simulink model "pathFollowingWithObstacleAvoidance"  (R2020a)
settings: Solver=FixedStepDiscrete  StartTime=0.0  StopTime=inf  FixedStep=0.001  RelTol=1e-3
model workspace (MAT data in the model file):
  SL_ROS_VariableLengthArrays_MaxSizes.CommonInfo.ArrayTruncateAction = 'EmitWarning'
  SL_ROS_VariableLengthArrays_MaxSizes.MsgTypeMap = containers.Map
  SL_ROS_VariableLengthArrays_MaxSizes.MsgTypeMap.serialization.keys = {'sensor_msgs/LaserScan'}
  SL_ROS_VariableLengthArrays_MaxSizes.MsgTypeMap.serialization.values{1}(1).PropertyName = 'Intensities'
  SL_ROS_VariableLengthArrays_MaxSizes.MsgTypeMap.serialization.values{1}(1).DataType = 'single'
  SL_ROS_VariableLengthArrays_MaxSizes.MsgTypeMap.serialization.values{1}(1).MaxLength = 360
  SL_ROS_VariableLengthArrays_MaxSizes.MsgTypeMap.serialization.values{1}(2).PropertyName = 'Ranges'
  SL_ROS_VariableLengthArrays_MaxSizes.MsgTypeMap.serialization.values{1}(2).DataType = 'single'
  SL_ROS_VariableLengthArrays_MaxSizes.MsgTypeMap.serialization.values{1}(2).MaxLength = 360
  SL_ROS_VariableLengthArrays_MaxSizes.MsgTypeMap.serialization.uniformity = 0
  SL_ROS_VariableLengthArrays_MaxSizes.MsgTypeMap.serialization.keyType = 'char'
  SL_ROS_VariableLengthArrays_MaxSizes.MsgTypeMap.serialization.valueType = 'any'
undefined symbols (not defined in the file): Angular, Linear
libraries: robotlib x4, robotalgslib x2, sharedtransform x1, simulink x1
settings Model: Creator=Zozo  LastModifiedBy=Zozo
settings OptimizationCC: EnhancedBackFolding=on  PassReuseOutputArgsAs=Individual arguments  ZeroExternalMemoryAtStartup=off  ZeroInternalMemoryAtStartup=off  MaxStackSize=64  OptimizeBlockOrder=speed  DifferentSizesBufferReuse=on  OptimizationCustomize=off  EfficientTunableParamExpr=on
settings DebuggingCC: ParameterTunabilityLossMsg=error
settings HardwareCC: ProdBitPerPointer=32  ProdBitPerSizeT=32  ProdBitPerPtrDiffT=32  ProdLargestAtomicFloat=None  ProdIntDivRoundTo=Undefined  ProdEndianess=Unspecified  ProdWordSize=32  ProdHWDeviceType=Generic->Unspecified (assume 32-bit Generic)
settings SFSimCC: MATLABDynamicMemAlloc=off
settings RTWCC: SystemTargetFile=ert.tlc  HardwareBoard=Robot Operating System (ROS)  TemplateMakefile=ert_default_tmf  Toolchain=Catkin  TargetLang=C++
settings CodeAppCC: ForceParamTrailComments=on  IgnoreCustomStorageClasses=off  OperatorAnnotations=on  SimulinkDataObjDesc=on  SFDataObjDesc=on  InsertBlockDesc=on

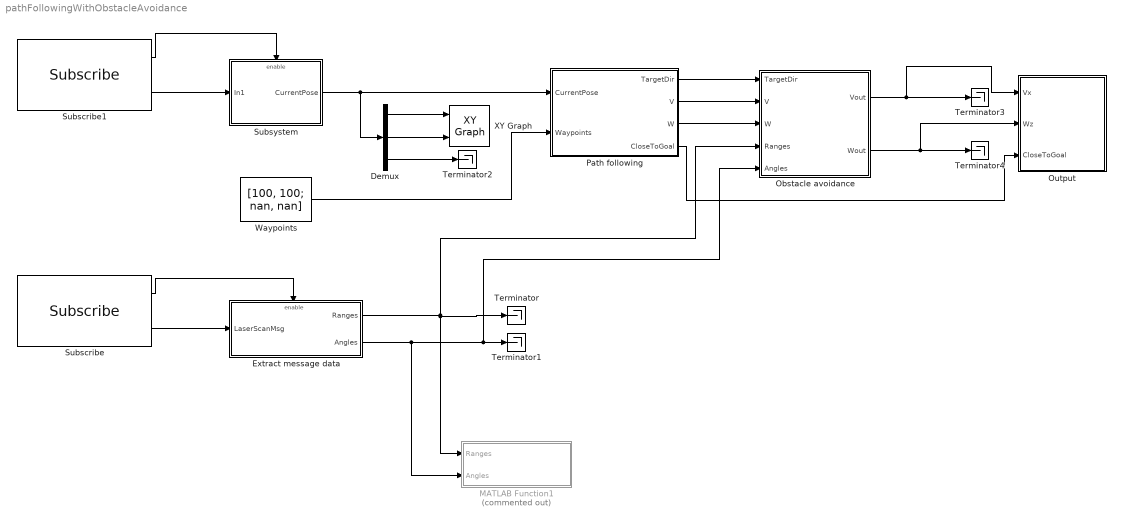
== system pathFollowingWithObstacleAvoidance ==
  Demux : Demux  Outputs=3
  Extract message data : Subsystem
  MATLAB Function1 : MATLAB Function  Commented=on  TreatAsAtomicUnit=on
  Obstacle avoidance : Subsystem
  Output : Subsystem
  Path following : Subsystem
  Subscribe : robotlib/Subscribe  topicSource=Select from ROS network  topic=/lidar2Dscan  messageType=sensor_msgs/LaserScan  sampleTime=-1  messageQueueLength=1
  Subscribe1 : robotlib/Subscribe  topicSource=Select from ROS network  topic=/mavros/local_position/pose  messageType=geometry_msgs/PoseStamped  sampleTime=-1  messageQueueLength=1
  Subsystem : Subsystem
  Terminator{,1..4} (5 alike) : Terminator
  Waypoints : Constant  Value=[100, 100; nan, nan]  OutDataTypeStr=double
  XY Graph : simulink/Sinks/XY Graph  xmin=-10  xmax=30  ymin=-10  ymax=10  st=-1
  wires:
  Subscribe/2 -> Extract message data/1(LaserScanMsg)
  Subscribe/1 -> Extract message data/Enable
  Extract message data/2(Angles) -> Obstacle avoidance/5(Angles), Terminator1/1, MATLAB Function1/2(Angles)
  Extract message data/1(Ranges) -> Terminator/1, MATLAB Function1/1(Ranges), Obstacle avoidance/4(Ranges)
  Subscribe1/2 -> Subsystem/1(In1)
  Subscribe1/1 -> Subsystem/Enable
  Demux/2 -> XY Graph/2
  Demux/1 -> XY Graph/1
  Demux/3 -> Terminator2/1
  Subsystem/1(CurrentPose) -> Path following/1(CurrentPose), Demux/1
  Waypoints/1 -> Path following/2(Waypoints)
  Path following/3(W) -> Obstacle avoidance/3(W)
  Path following/2(V) -> Obstacle avoidance/2(V)
  Path following/1(TargetDir) -> Obstacle avoidance/1(TargetDir)
  Obstacle avoidance/1(Vout) -> Output/1(Vx), Terminator3/1
  Obstacle avoidance/2(Wout) -> Output/2(Wz), Terminator4/1
  Path following/4(CloseToGoal) -> Output/3(CloseToGoal)

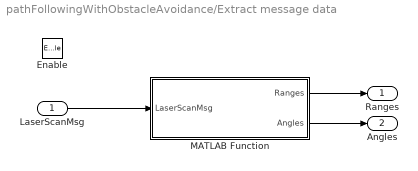
== system pathFollowingWithObstacleAvoidance/Extract message data ==
  LaserScanMsg : Inport
  Enable : EnablePort
  MATLAB Function : MATLAB Function  TreatAsAtomicUnit=on
  Ranges : Outport
  Angles : Outport  Port=2
  wires:
  MATLAB Function/1(Ranges) -> Ranges/1
  MATLAB Function/2(Angles) -> Angles/1
  LaserScanMsg/1 -> MATLAB Function/1(LaserScanMsg)

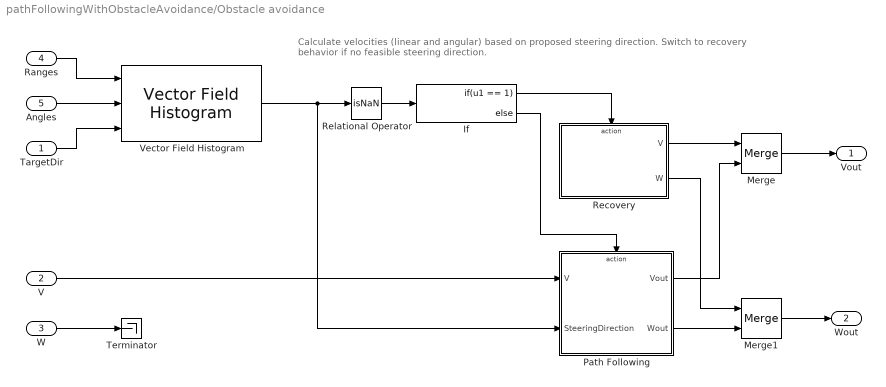
== system pathFollowingWithObstacleAvoidance/Obstacle avoidance ==
  note: Calculate velocities (linear and angular) based on proposed steering direction.
      | 				Switch to recovery behavior if no feasible steering direction.
  TargetDir : Inport
  V : Inport  Port=2
  W : Inport  Port=3
  Ranges : Inport  Port=4
  Angles : Inport  Port=5
  If : If  IfExpression=u1 == 1
  Merge : Merge
  Merge1 : Merge
  Path Following : Subsystem  TreatAsAtomicUnit=on
  Recovery : Subsystem  TreatAsAtomicUnit=on
  Relational Operator : RelationalOperator  Operator=isNaN  OutDataTypeStr=boolean  RndMeth=Simplest
  Terminator : Terminator
  Vector Field Histogram : robotalgslib/Vector Field Histogram  NumAngularSectors=180  DistanceLimits=[0.5, 4]  HistogramThresholds=[3, 10]  RobotRadius=0.25  SafetyDistance=0.25  MinTurningRadius=0.1  SimulateUsing=Code generation  TargetDirectionWeight=5  CurrentDirectionWeight=2  PreviousDirectionWeight=2
      settings: SourceProductBaseCode=RO
  Vout : Outport
  Wout : Outport  Port=2
  wires:
  V/1 -> Path Following/1(V)
  Vector Field Histogram/1 -> Path Following/2(SteeringDirection), Relational Operator/1
  Relational Operator/1 -> If/1
  Angles/1 -> Vector Field Histogram/2
  Merge/1 -> Vout/1
  TargetDir/1 -> Vector Field Histogram/3
  Ranges/1 -> Vector Field Histogram/1
  If/1 -> Recovery/Action
  If/2 -> Path Following/Action
  Recovery/2(W) -> Merge1/1
  Path Following/2(Wout) -> Merge1/2
  Recovery/1(V) -> Merge/1
  Path Following/1(Vout) -> Merge/2
  Merge1/1 -> Wout/1
  W/1 -> Terminator/1

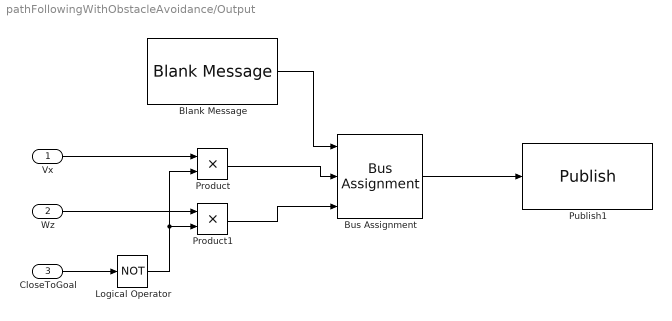
== system pathFollowingWithObstacleAvoidance/Output ==
  Vx : Inport
  Wz : Inport  Port=2
  CloseToGoal : Inport  Port=3
  Blank Message : robotlib/Blank Message  messageClass=Message  entityType=geometry_msgs/Twist  messageType=geometry_msgs/Twist  SampleTime=0
  Bus Assignment : BusAssignment  DialogController=Simulink.DDGSource_BusAssignment  AssignedSignals=Linear.X,Angular.Z
  Logical Operator : Logic  Operator=NOT  AllPortsSameDT=off  OutDataTypeStr=boolean
  Product : Product
  Product1 : Product
  Publish1 : robotlib/Publish  topicSource=Specify your own  topic=/simulink/cmd_vel  messageType=geometry_msgs/Twist  messageQueueLength=105
  wires:
  Bus Assignment/1 -> Publish1/1
  Blank Message/1 -> Bus Assignment/1
  Logical Operator/1 -> Product1/2, Product/2
  Product1/1 -> Bus Assignment/3
  CloseToGoal/1 -> Logical Operator/1
  Vx/1 -> Product/1
  Wz/1 -> Product1/1
  Product/1 -> Bus Assignment/2

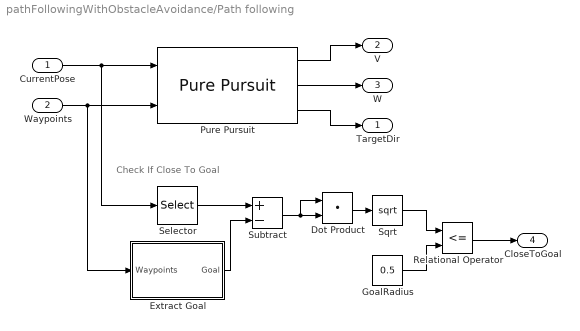
== system pathFollowingWithObstacleAvoidance/Path following ==
  note: Check If Close To Goal
  CurrentPose : Inport
  Waypoints : Inport  Port=2
  " Extract Goal" : MATLAB Function  TreatAsAtomicUnit=on
  Dot Product : DotProduct  InputSameDT=on  OutDataTypeStr=Inherit: Inherit via internal rule
  GoalRadius : Constant  Value=0.5
  Pure Pursuit : robotalgslib/Pure Pursuit  DesiredLinearVelocity=0.5  MaxAngularVelocity=1.0  LookaheadDistance=2.0  TargetDirPort=on  SimulateUsing=Code generation
      settings: SourceProductBaseCode=RO
  Relational Operator : RelationalOperator  Operator=<=  OutDataTypeStr=boolean  RndMeth=Simplest
  Selector : Selector  InputPortWidth=3  IndexOptions=Index vector (dialog)  Indices=[1 2]  OutputSizes=1
  Sqrt : Sqrt  SaturateOnIntegerOverflow=on
  Subtract : Sum  Inputs=+-
  TargetDir : Outport
  V : Outport  Port=2
  W : Outport  Port=3
  CloseToGoal : Outport  Port=4
  wires:
  Pure Pursuit/3 -> TargetDir/1
  Pure Pursuit/2 -> W/1
  Pure Pursuit/1 -> V/1
  " Extract Goal"/1(Goal) -> Subtract/2
  Waypoints/1 -> " Extract Goal"/1(Waypoints), Pure Pursuit/2
  CurrentPose/1 -> Selector/1, Pure Pursuit/1
  Relational Operator/1 -> CloseToGoal/1
  GoalRadius/1 -> Relational Operator/2
  Selector/1 -> Subtract/1
  Dot Product/1 -> Sqrt/1
  Sqrt/1 -> Relational Operator/1
  Subtract/1 -> Dot Product/1, Dot Product/2

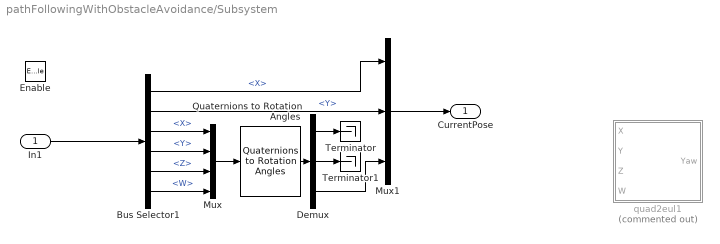
== system pathFollowingWithObstacleAvoidance/Subsystem ==
  In1 : Inport
  Enable : EnablePort
  Bus Selector1 : BusSelector  OutputSignals=Pose.Position.X,Pose.Position.Y,Pose.Orientation.X,Pose.Orientation.Y,Pose.Orientation.Z,Pose.Orientation.W
  Demux : Demux  Outputs=3
  Mux : Mux
  Mux1 : Mux  Inputs=3
  Quaternions to Rotation Angles : sharedtransform/Quaternions to Rotation Angles  rotationOrder=ZYX  aMode=aMode
      settings: SourceProductBaseCode=AE,PW,MT,VE,VP
  Terminator : Terminator
  Terminator1 : Terminator
  quad2eul1 : MATLAB Function  Commented=on  TreatAsAtomicUnit=on
  CurrentPose : Outport
  wires:
  Bus Selector1/4 -> Mux/2  "<Y>"
  Bus Selector1/3 -> Mux/1  "<X>"
  Bus Selector1/2 -> Mux1/2  "<Y>"
  Demux/3 -> Mux1/3
  Mux1/1 -> CurrentPose/1
  Bus Selector1/6 -> Mux/4  "<W>"
  Bus Selector1/1 -> Mux1/1  "<X>"
  In1/1 -> Bus Selector1/1
  Bus Selector1/5 -> Mux/3  "<Z>"
  Mux/1 -> Quaternions to Rotation Angles/1
  Quaternions to Rotation Angles/1 -> Demux/1
  Demux/1 -> Terminator/1
  Demux/2 -> Terminator1/1

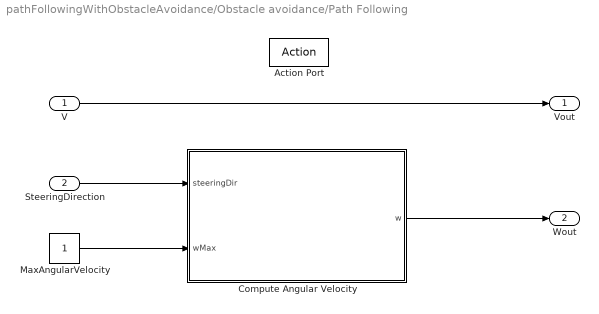
== system pathFollowingWithObstacleAvoidance/Obstacle avoidance/Path Following ==
  V : Inport
  SteeringDirection : Inport  Port=2
  Action Port : ActionPort  ActionPortLabel=else
  Compute Angular Velocity : MATLAB Function  TreatAsAtomicUnit=on
  MaxAngularVelocity : Constant
  Vout : Outport
  Wout : Outport  Port=2
  wires:
  V/1 -> Vout/1
  MaxAngularVelocity/1 -> Compute Angular Velocity/2(wMax)
  SteeringDirection/1 -> Compute Angular Velocity/1(steeringDir)
  Compute Angular Velocity/1(w) -> Wout/1

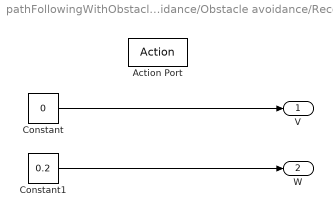
== system pathFollowingWithObstacleAvoidance/Obstacle avoidance/Recovery ==
  Action Port : ActionPort  ActionPortLabel=if(u1 == 1)
  Constant : Constant  Value=0
  Constant1 : Constant  Value=0.2
  V : Outport
  W : Outport  Port=2
  wires:
  Constant1/1 -> W/1
  Constant/1 -> V/1

== matlab function pathFollowingWithObstacleAvoidance/Subsystem/quad2eul1 ==
  data: X input; Yaw output; Y input; Z input; W input
function Yaw = quat2eulBlk(X, Y, Z, W)
%#codegen

eularAngles = quat2eul([W, X, Y, Z]);
Yaw = eularAngles(1);

== matlab function pathFollowingWithObstacleAvoidance/MATLAB Function1 ==
  data: Ranges input; Angles input
function plotLaser(Ranges, Angles)
coder.extrinsic('polarplot');
persistent p;
if isempty(p)
    p = polarplot(0, 0, '.');
    set(gca, 'ThetaZeroLocation', 'top', 'ThetaLim', [-180 180], ...
        'RAxisLocation', 0, 'RLim', [0 10]);
end
if ishandle(p)
    set(p, 'ThetaData', Angles);
    set(p, 'RData', Ranges);
    drawnow limitrate;
end

== matlab function pathFollowingWithObstacleAvoidance/Extract message data/MATLAB Function ==
  data: LaserScanMsg input; Ranges output; Angles output
function [Ranges, Angles] = ExtractRangeData(LaserScanMsg)
%#codegen

% Extract Range information
Ranges = double(LaserScanMsg.Ranges);

% Construct Angles vector using AngleMin and AngleIncrement from sensor
% reading.
angMin = double(LaserScanMsg.AngleMin);
angMax = double(LaserScanMsg.AngleMax);
numel(Ranges)
rawAngles = linspace(angMax, angMin, numel(Ranges));

% Wrap the angles to the (-pi,pi] interval.
Angles = robotics.internal.wrapToPi(double(rawAngles));

== matlab function pathFollowingWithObstacleAvoidance/Path following/ Extract Goal ==
  data: Waypoints input; Goal output
function Goal = extractGoal(Waypoints)
%#codegen
b = isnan(Waypoints);
[rows,~] = find(b);
ridx = setdiff(1:size(Waypoints,1), sort(rows));
Goal = [Waypoints(ridx(end), 1) Waypoints(ridx(end), 2)];

== matlab function pathFollowingWithObstacleAvoidance/Obstacle avoidance/Path Following/Compute Angular Velocity ==
  data: steeringDir input; w output; wMax input
function w = exampleHelperComputeAngularVelocity(steeringDir, wMax)
%EXAMPLEHELPERCOMPUTEANGULARVELOCITY Compute angular velocity
%   W = exampleHelperComputeAngularVelocity(STEERINGDIR)
%   returns the angular velocity W for a differential drive robot in radians
%   per second for a given steering direction STEERINGDIR in the robot's
%   coordinate frame in radians.
%
%   W = exampleHelperComputeAngularVelocity(STEERINGDIR, WMAX)
%   returns the angular velocity W for a differential drive robot in radians
%   per second for a given steering direction STEERINGDIR in the robot's
%   coordinate frame in radians and maximum angular velocity WMAX in
%   radians per second. The output angular velocity is saturated based on
%   the WMAX.
%
%   Example:
%       
%       w = exampleHelperComputeAngularVelocity(0.2, 1);

% Copyright 2015 The MathWorks, Inc.

%#codegen
%#ok<*EMCA>

% Allow variable input arguments
if nargin == 1   
    wMax = inf;
end

validateattributes(steeringDir, {'double'},{'real'},...
    'exampleHelperComputeAngularVelocity', 'STEERINGDIR', 1);
validateattributes(wMax, {'double'},{'real', 'positive'},...
    'exampleHelperComputeAngularVelocity', 'WMAX', 2);

% Computing in robot's coordinate frame
curPose = [0 0 0];

% The following computation is similar to robotics.PurePursuit
lookaheadPoint = [cos(steeringDir), sin(steeringDir)];
slope = atan2((lookaheadPoint(2) - curPose(2)), ...
    (lookaheadPoint(1) - curPose(1)));
alpha = angdiff(curPose(3), slope);

% Angular velocity command for a differential drive robot is
% equal to the desired curvature to be followed by the robot.

w = (2*sin(alpha));

% Pick a constant rotation when robot is facing in the opposite
% direction of the path
if abs(abs(alpha) - pi) < 1e-12
    w = sign(w)*1;
end

if abs(w) > wMax
    w = sign(w)*wMax;
end

end
